simulink model "TesteParaProjetoComBlocoPilotoComPneus"  (R2024b)
settings: Solver=VariableStepAuto  StartTime=0.0  StopTime=100  RelTol=1e-3
values from neighbouring files (symbols this model uses):
  s = size(xRef)    [CodigoSimulacao2D.m]
undefined symbols (not defined in the file or in its folder): C1, C2, C3, EV
libraries: autolibshared x5, autolibmappedmotor x2, slpidlib x1, vehdynlibviscommon x1, vehdynlibscenariocommon x1, vehdynlibsteering x1, vehdynlibdriver x1
(part 1 of 4)
settings Model: SimulationMode=accelerator  Creator=João Gabriel  LastModifiedBy=Pedro Lemos

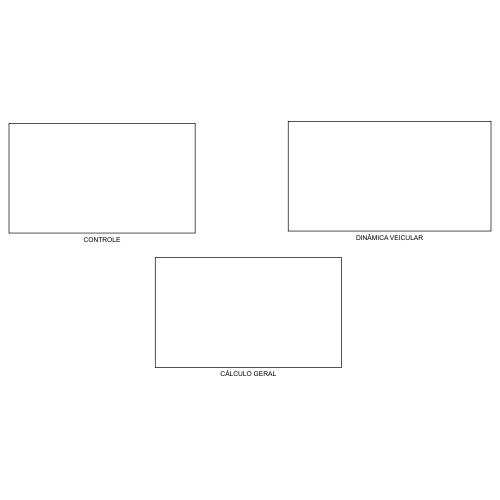
[thumbnail: Simulink's stored preview of the top-level diagram]
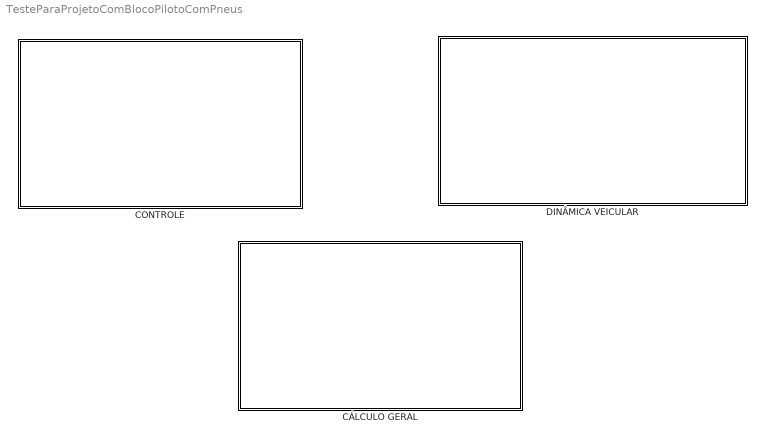
== system TesteParaProjetoComBlocoPilotoComPneus ==
  CONTROLE : Subsystem
  CÁLCULO GERAL : Subsystem
  DINÂMICA VEICULAR : Subsystem

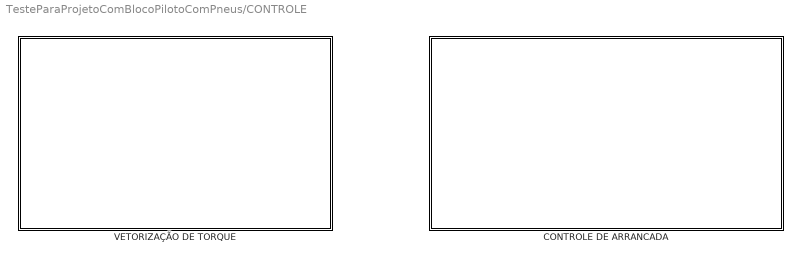
== system TesteParaProjetoComBlocoPilotoComPneus/CONTROLE ==
  "CONTROLE DE ARRANCADA " : Subsystem
  "VETORIZAÇÃO DE TORQUE " : Subsystem

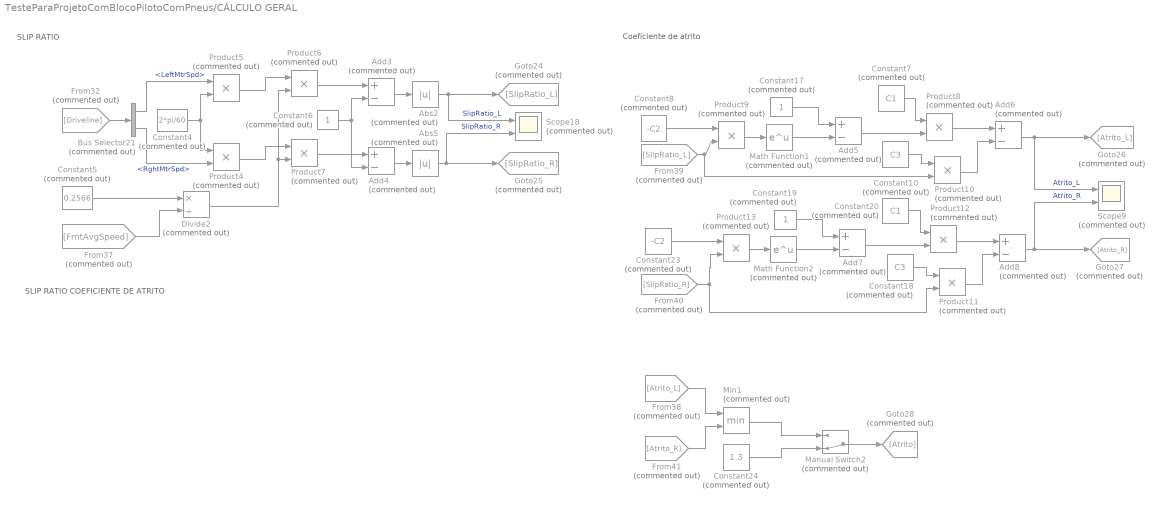
== system TesteParaProjetoComBlocoPilotoComPneus/CÁLCULO GERAL ==
  note: SLIP RATIO
  note: Coeficiente de atrito
  note: SLIP RATIO
      |
      | COEFICIENTE DE ATRITO
  Abs2 : Abs  Commented=on  SaturateOnIntegerOverflow=off
  Abs5 : Abs  Commented=on  SaturateOnIntegerOverflow=off
  Add{3..8} (6 alike) : Sum  Commented=on  Inputs=+-
  Bus Selector21 : BusSelector  Commented=on  OutputSignals=LeftMtrSpd,RghtMtrSpd
  Constant10 : Constant  Commented=on  Value=C3
  Constant17 : Constant  Commented=on
  Constant18 : Constant  Commented=on  Value=C3
  Constant19 : Constant  Commented=on
  Constant20 : Constant  Commented=on  Value=C1
  Constant23 : Constant  Commented=on  Value=-C2
  Constant24 : Constant  Commented=on  Value=1.3
  Constant4 : Constant  Commented=on  Value=2*pi/60
  Constant5 : Constant  Commented=on  Value=0.2566
  Constant6 : Constant  Commented=on
  Constant7 : Constant  Commented=on  Value=C1
  Constant8 : Constant  Commented=on  Value=-C2
  Divide2 : Product  Commented=on  Inputs=*/
  From32 : From  Commented=on  GotoTag=Driveline
  From37 : From  Commented=on  GotoTag=FrntAvgSpeed
  From38 : From  Commented=on  GotoTag=Atrito_L
  From39 : From  Commented=on  GotoTag=SlipRatio_L
  From40 : From  Commented=on  GotoTag=SlipRatio_R
  From41 : From  Commented=on  GotoTag=Atrito_R
  Goto24 : Goto  Commented=on  GotoTag=SlipRatio_L
  Goto25 : Goto  Commented=on  GotoTag=SlipRatio_R
  Goto26 : Goto  Commented=on  GotoTag=Atrito_L
  Goto27 : Goto  Commented=on  GotoTag=Atrito_R
  Goto28 : Goto  Commented=on  GotoTag=Atrito
  Manual Switch2 : ManualSwitch  Commented=on  CurrentSetting=0
  Math Function1 : Math  Commented=on
  Math Function2 : Math  Commented=on
  Min1 : MinMax  Commented=on  Inputs=2
  Product{4..13} (10 alike) : Product  Commented=on
  Scope18 : Scope  Commented=on  NumInputPorts=2
  Scope9 : Scope  Commented=on  NumInputPorts=2
  wires:
  Constant6/1 -> Add3/2, Add4/2
  From32/1 -> Bus Selector21/1
  Add6/1 -> Scope9/1, Goto26/1  "Atrito_L"
  Abs2/1 -> Scope18/1, Goto24/1  "SlipRatio_L"
  Constant4/1 -> Product5/2, Product4/1
  Constant7/1 -> Product8/1
  Constant19/1 -> Add7/1
  Constant24/1 -> Manual Switch2/2
  Constant23/1 -> Product13/1
  Add4/1 -> Abs5/1
  Add3/1 -> Abs2/1
  Product11/1 -> Add8/2
  Abs5/1 -> Scope18/2, Goto25/1  "SlipRatio_R"
  Product12/1 -> Add8/1
  Product4/1 -> Product7/1
  Product10/1 -> Add6/2
  Product8/1 -> Add6/1
  Math Function2/1 -> Add7/2
  Bus Selector21/1 -> Product5/1  "<LeftMtrSpd>"
  Add7/1 -> Product12/2
  From38/1 -> Min1/1
  Constant10/1 -> Product10/1
  Math Function1/1 -> Add5/2
  Constant18/1 -> Product11/1
  From39/1 -> Product10/2, Product9/2
  Bus Selector21/2 -> Product4/2  "<RghtMtrSpd>"
  Add8/1 -> Scope9/2, Goto27/1  "Atrito_R"
  Product9/1 -> Math Function1/1
  From37/1 -> Divide2/2
  Min1/1 -> Manual Switch2/1
  Constant8/1 -> Product9/1
  Constant17/1 -> Add5/1
  From41/1 -> Min1/2
  Constant5/1 -> Divide2/1
  Divide2/1 -> Product6/2, Product7/2
  Product13/1 -> Math Function2/1
  Constant20/1 -> Product12/1
  Product7/1 -> Add4/1
  Product5/1 -> Product6/1
  Add5/1 -> Product8/2
  From40/1 -> Product13/2, Product11/2
  Product6/1 -> Add3/1
  Manual Switch2/1 -> Goto28/1
